simulink model "CellVoltageDiagnostics_HIL_Test_Automation"  (R2022b)
settings: Solver=FixedStepDiscrete  StartTime=0.0  StopTime=100  FixedStep=0.001  RelTol=1e-3  EnableMultiTasking=on
PreLoadFcn:
  | ts = 0.1
libraries: fl_lib x9, nesl_utility x9, speedgoatlib_IO133 x2, speedgoatlib_PIL x1, BatteryPack_lib x1
settings Model: DataDictionary=Shared_DD_TMS570.sldd  sg_rtwmakecfg_data=_sglibc__PIL_HWD__Pilpxi_  SimulationMode=external  Creator=cpatel  LastModifiedBy=mathieu.lu-dac
settings SolverCC: ConcurrentTasks=on  AlgebraicLoopSolver=TrustRegion  PositivePriorityOrder=on  AutoInsertRateTranBlk=on  InsertRTBMode=Never (minimum delay)
settings DataIOCC: SaveFormat=StructureWithTime  SaveOutput=off  SignalLogging=off  DSMLogging=off  SaveTime=off  SignalLoggingName=logsOut
settings OptimizationCC: BlockReduction=off  BooleanDataType=off  OptimizeBlockIOStorage=off  BufferReuse=off  GlobalBufferReuse=off  ExpressionFolding=off  LocalBlockOutputs=off  InitFltsAndDblsToZero=on  OptimizeDataStoreBuffers=off  BusAssignmentInplaceUpdate=off
settings DebuggingCC: SaveWithParameterizedLinksMsg=none  CheckExecutionContextPreStartOutputMsg=on  SignalResolutionControl=TryResolveAllWithWarning  TasksWithSamePriorityMsg=none  UnconnectedInputMsg=warning  UnconnectedOutputMsg=warning  UnconnectedLineMsg=warning  SFUnexpectedBacktrackingDiag=warning  SFNoUnconditionalDefaultTransitionDiag=warning  SFExecutionAtInitializationDiag=none  SFMachineParentedDataDiag=warning  ArithmeticOperatorsInVariantConditions=warning
settings HardwareCC: ProdBitPerLong=64  ProdLongLongMode=on  ProdHWDeviceType=Intel->x86-64 (Linux 64)
settings ModelReferenceCC: EnableRefExpFcnMdlSchedulingChecks=on  PropagateSignalLabelsOutOfModel=off
settings SFSimCC: SimUseLocalCustomCode=off  CustomCodeUndefinedFunction=UseInterfaceOnly
settings RTWCC: Description=Simulink Real-Time  SystemTargetFile=slrealtime.tlc  TemplateMakefile=slrealtime_default_tmf  RTWVerbose=off  RTWUseLocalCustomCode=off  Toolchain=Simulink Real-Time Toolchain  BuildConfiguration=Faster Runs  CodeExecutionProfiling=on  TargetLang=C++  DLArmComputeVersion=19.05
settings CodeAppCC: StateflowObjectComments=on
settings SimulinkRealTimeTargetCC: UseGCCFastMath=on
settings ConfigComp: CovMetricSettings=dw  CovSaveCumulativeToWorkspaceVar=on  CovSaveSingleToWorkspaceVar=on  CovExternalEMLEnable=off  CovSFcnEnable=off

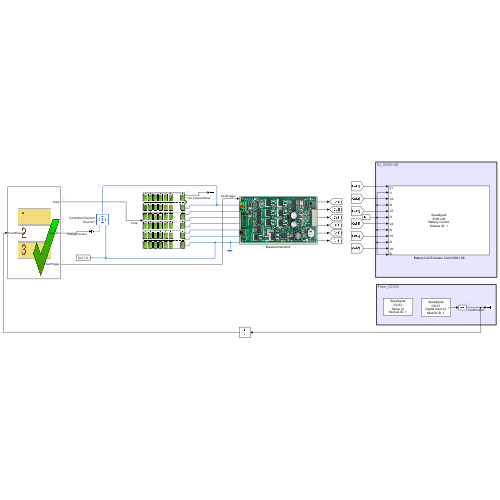
[thumbnail: Simulink's stored preview of the top-level diagram]
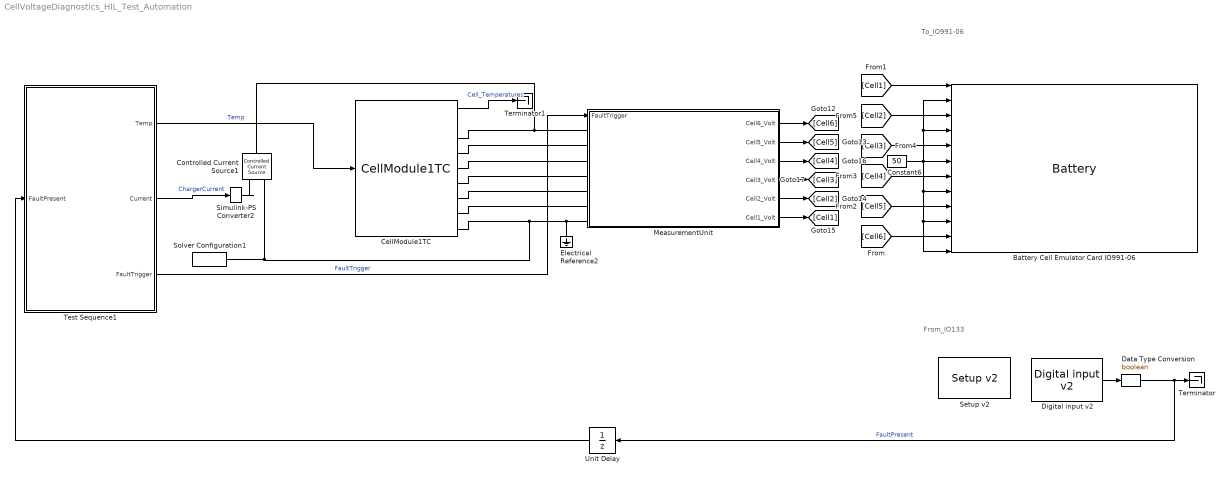
== system CellVoltageDiagnostics_HIL_Test_Automation ==
  note: To_IO991-06
  note: From_IO133
  Battery Cell Emulator Card IO991-06 : speedgoatlib_PIL/Battery  id=1  card_type=IO991-06 (6 channels, 0-7V output, 300mA source, 100mA sink)  channel_vector=[1,2,3,4,5,6]  init_enable_vector=ones(1,6)  reset_enable_vector=ones(1,6)  init_voltage_vector=3.6*ones(1,6)  reset_voltage_vector=ones(1,6)  init_current_vector=[0]  reset_current_vector=[0]  show_input_enable=off  show_output=off  ts=ts  slot=[6,15]  VendorID=0  SubVendorID=0  DeviceID=0  SubDeviceID=0  category=1  NumCh=0  MinVout=0  MaxVout=0  MinIsink=0  MaxIsink=0  mask(IOPIL_battery){}
      settings: SourceProductName=Simulink Real-Time: Speedgoat I/O Blockset
  CellModule1TC : BatteryPack_lib/CellModule1TC  SystemSampleTime=-1  VariantActivationTime=update diagram  Latency=0  AutoFrameSizeCalculation=off
      mask Display:
      | % This is a new mask on top of the base mask.
      | % Use "View base mask" link below to see the base mask.
      | image('BatteryPack.png');
  Constant6 : Constant  Value=50
  Controlled Current Source1 : fl_lib/Electrical/Electrical Sources/Controlled Current Source
      settings: LogSimulationData=on
  Data Type Conversion : DataTypeConversion  OutDataTypeStr=boolean  SaturateOnIntegerOverflow=off  RndMeth=Floor
  "Digital input v2 " : speedgoatlib_IO133/Digital input v2   parModuleId=1  parSampleTime=0.1  parPciSlot=-1  parDiChannels=1
      settings: SourceProductName=Simulink Real-Time: Speedgoat I/O Blockset
  Electrical Reference2 : fl_lib/Electrical/Electrical Elements/Electrical Reference
  MeasurementUnit : Subsystem
      mask Display: image('TCU.png');
  "Setup v2 " : speedgoatlib_IO133/Setup v2   parPciSlot=-1  parModuleId=1  parInterModuleSync=None  parConvClockBaseRate=20MHz  parConvClock1Divider=20000  parConvClock2Divider=20000  parFrameTriggerEnable=off  parFrameTriggerDivider=10  parConvClock1BaseRate=1  parConvClock2BaseRate=1  parFrameTriggerClock=1  parAdcChannels=[]  parAdcRange1=+-5V  parAdcRange2=+-5V  parAdcVoltageRange=[1 1]  parAdcOversampling1=None  parAdcOversampling2=None  parAdcOversamplRate=[1 1]  parAdcAutoCorrection=on  parAdcContSampling=off  parAdcDmaEnable=off  parAdcDmaClock=Clock 1  parAdcFrameSize_=100  parAdcSampleTime_=-1  parAdcActiveDmaDevices=[1 1]  parAdcFrameTriggerEnable=0  parAdcFrameSize=100  parAdcSampleTime=0.1  parDacChannels=[1]  parDacInitValues=0  parDacReset=1  parDacRange1=0-5V  parDacRange2=0-5V  parDacRange3=0-5V  parDacRange4=0-5V  parDacRange5=0-5V  parDacRange6=0-5V  parDacRange7=0-5V  parDacRange8=0-5V  parDacVoltageRange=[1 1 1 1 1 1 1 1]  parDacAutoCorrection=on  parDacSyncOut=on  parDacDmaEnable=off  parDacDmaLatency=Until next frame  parDacDmaClock=Clock 1  parDacFrameSize_=100  parDacSampleTime_=-1  parDacActiveDmaDevices=[1 1]  parDacFrameTriggerEnable=0  parDacFrameSize=100  parDacSampleTime=0.1  parDoChannels=[]  parDoInitValues=0  parDoReset=0  parDiChannels=[1]  parDiDebounceEnable=off  parDiDebounceTime=0  parDiDebounceValue=0  parDioPullRefFront=Pull-up 3.3V  parDioPullRefRear=Floating
      settings: SourceProductName=Simulink Real-Time: Speedgoat I/O Blockset
  Simulink-PS Converter2 : nesl_utility/Simulink-PS Converter  PhysicalDomain=network_engine_domain  SubClassName=ps_input  LeftPortType=input  RightPortType=output  PseudoPeriodic=off  Frequencies=[]  NoiseDistribution=none  NoiseParameters=[]  Unit=1  AffineConversion=off  FilteringAndDerivatives=zero  SimscapeFilterOrder=1  InputFilterTimeConstant=0.001  UdotUserProvided=1
  Solver Configuration1 : nesl_utility/Solver Configuration  PhysicalDomain=network_engine_domain  SubClassName=solver  LeftPortType=input  RightPortType=generic  Tones=[]  Harmonics=[]  SimulateNoise=off  Profile=off  UseLocalSampling=off  EnableSwitchedLinearOptims=on  FrequencyDomain=off  UseCCode=off  RelTol=0.001  AbsTol=1e-06  MinStep=1e-09  ToWorkspace=off  RevertToSquareIcSolve=off  NumHomotopyIterations=100  PhasorMode=off  PhasorModeNumHarmonics=1  ConsistencySolver=NEWTON_FTOL  IndexReductionMethod=DerivativeReplacement  DoDC=off  ResidualTolerance=1e-09  ConsistencyTolSource=GLOBAL  ConsistencyAbsTol=0.001  ConsistencyRelTol=0.001  ConsistencyTolFactor=0.001  UseLocalSolver=on  LocalSolverChoice=NE_BACKWARD_EULER_ADVANCER  ResolveIndetEquations=on  FunctionEvalNumThread=1  LocalSolverSampleTime=ts  DoFixedCost=on  MaxNonlinIter=3  MaxModeIter=2  ComputeImpulses=off  ImpulseIterations=2  LinearAlgebra=auto  LinearAlgebraNumThread=0  EquationFormulation=NE_TIME_EF  DelaysMemoryBudget=1024  AutomaticFiltering=off  FilteringTimeConstant=0.001  PartitionStorageMethod=AS_NEEDED  PartitionMemoryBudget=1024  PartitionMethod=FAST
  Terminator : Terminator
  Terminator1 : Terminator
  Test Sequence1 : Test Sequence  TreatAsAtomicUnit=on
  Unit Delay : UnitDelay  SampleTime=-1  HasFrameUpgradeWarning=on
  wires:
  Data Type Conversion/1 -> Unit Delay/1, Terminator/1  "FaultPresent"
  "Digital input v2 "/1 -> Data Type Conversion/1
  Constant6/1 -> Battery Cell Emulator Card IO991-06/2, Battery Cell Emulator Card IO991-06/4, Battery Cell Emulator Card IO991-06/6, Battery Cell Emulator Card IO991-06/12, Battery Cell Emulator Card IO991-06/10, Battery Cell Emulator Card IO991-06/8
  [Cell6] -> Battery Cell Emulator Card IO991-06/11
  [Cell1] -> Battery Cell Emulator Card IO991-06/1
  [Cell5] -> Battery Cell Emulator Card IO991-06/9
  [Cell4] -> Battery Cell Emulator Card IO991-06/7
  [Cell3] -> Battery Cell Emulator Card IO991-06/5
  [Cell2] -> Battery Cell Emulator Card IO991-06/3
  Unit Delay/1 -> Test Sequence1/1(FaultPresent)
  MeasurementUnit/6(Cell1_Volt) -> [Cell1]
  MeasurementUnit/5(Cell2_Volt) -> [Cell2]
  CellModule1TC/1 -> Terminator1/1  "Cell_Temperatures"
  MeasurementUnit/3(Cell4_Volt) -> [Cell4]
  Test Sequence1/3(FaultTrigger) -> MeasurementUnit/1(FaultTrigger)  "FaultTrigger"
  Test Sequence1/2(Current) -> Simulink-PS Converter2/1  "ChargerCurrent"
  MeasurementUnit/2(Cell5_Volt) -> [Cell5]
  Test Sequence1/1(Temp) -> CellModule1TC/1  "Temp"
  MeasurementUnit/1(Cell6_Volt) -> [Cell6]
  MeasurementUnit/4(Cell3_Volt) -> [Cell3]
  connections:
  CellModule1TC/RConn7 -- Solver Configuration1/RConn1 -- Controlled Current Source1/RConn2 -- Electrical Reference2/LConn1 -- MeasurementUnit/LConn7
  MeasurementUnit/LConn1 -- CellModule1TC/RConn1 -- Controlled Current Source1/LConn1
  CellModule1TC/RConn4 -- MeasurementUnit/LConn4
  CellModule1TC/RConn3 -- MeasurementUnit/LConn3
  CellModule1TC/RConn6 -- MeasurementUnit/LConn6
  Simulink-PS Converter2/RConn1 -- Controlled Current Source1/RConn1
  CellModule1TC/RConn2 -- MeasurementUnit/LConn2
  CellModule1TC/RConn5 -- MeasurementUnit/LConn5

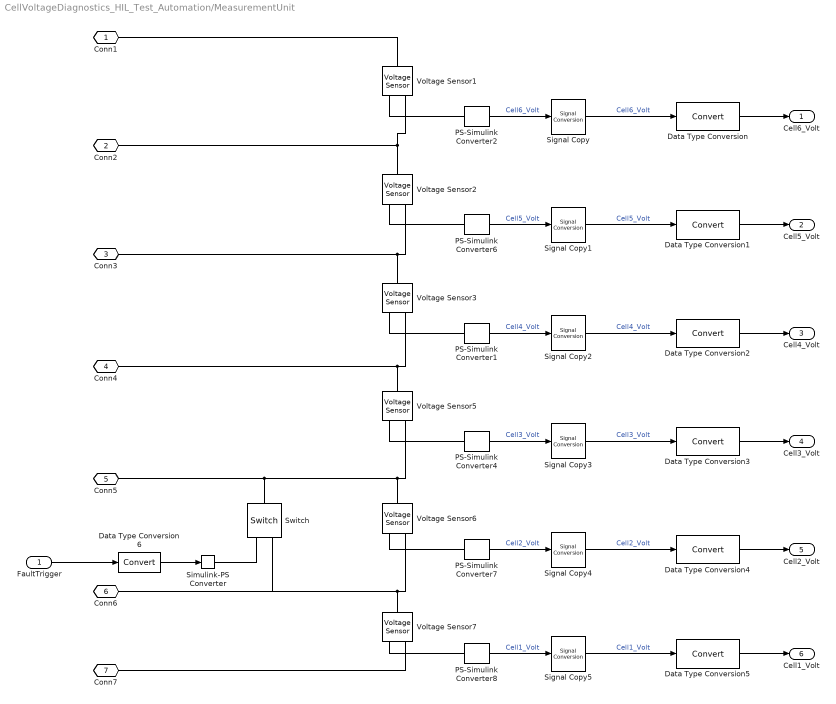
== system CellVoltageDiagnostics_HIL_Test_Automation/MeasurementUnit ==
  FaultTrigger : Inport
  Data Type Conversion{,1..6} (7 alike) : DataTypeConversion  SaturateOnIntegerOverflow=off  RndMeth=Floor
  PS-Simulink Converter{1..2,4,6..8} (6 alike) : nesl_utility/PS-Simulink Converter  PhysicalDomain=network_engine_domain  SubClassName=ps_output  LeftPortType=input  RightPortType=output  PseudoPeriodic=off  Frequencies=[]  VectorFormat=1-D array  Unit=V  AffineConversion=off
  Signal Copy{,1..5} (6 alike) : SignalConversion  OverrideOpt=off
  Simulink-PS Converter : nesl_utility/Simulink-PS Converter  PhysicalDomain=network_engine_domain  SubClassName=ps_input  LeftPortType=input  RightPortType=output  PseudoPeriodic=off  Frequencies=[]  NoiseDistribution=none  NoiseParameters=[]  Unit=1  AffineConversion=off  FilteringAndDerivatives=provide  SimscapeFilterOrder=1  InputFilterTimeConstant=0.001  UdotUserProvided=0
  Switch : fl_lib/Electrical/Electrical Elements/Switch  R_closed=0.01 Ohm  G_open=1e-8 1/Ohm  Threshold=0.5  i_specify=off  i_priority=None  i=0 A  i_nominal_specify=off  i_nominal_unit=A  i_nominal_value=1  v_specify=off  v_priority=None  v=0 V  v_nominal_specify=off  v_nominal_unit=V  v_nominal_value=1
  Voltage Sensor{1..3,5..7} (6 alike) : fl_lib/Electrical/Electrical Sensors/Voltage Sensor
  Conn1 : PMIOPort  Side=Left
  Conn2 : PMIOPort  Port=2  Side=Left
  Conn3 : PMIOPort  Port=3  Side=Left
  Conn4 : PMIOPort  Port=4  Side=Left
  Conn5 : PMIOPort  Port=5  Side=Left
  Conn6 : PMIOPort  Port=6  Side=Left
  Conn7 : PMIOPort  Port=7  Side=Left
  Cell6_Volt : Outport  VectorParamsAs1DForOutWhenUnconnected=off
  Cell5_Volt : Outport  Port=2  VectorParamsAs1DForOutWhenUnconnected=off
  Cell4_Volt : Outport  Port=3  VectorParamsAs1DForOutWhenUnconnected=off
  Cell3_Volt : Outport  Port=4  VectorParamsAs1DForOutWhenUnconnected=off
  Cell2_Volt : Outport  Port=5  VectorParamsAs1DForOutWhenUnconnected=off
  Cell1_Volt : Outport  Port=6  VectorParamsAs1DForOutWhenUnconnected=off
  wires:
  PS-Simulink Converter1/1 -> Signal Copy2/1  "Cell4_Volt"
  PS-Simulink Converter7/1 -> Signal Copy4/1  "Cell2_Volt"
  PS-Simulink Converter2/1 -> Signal Copy/1  "Cell6_Volt"
  PS-Simulink Converter4/1 -> Signal Copy3/1  "Cell3_Volt"
  PS-Simulink Converter8/1 -> Signal Copy5/1  "Cell1_Volt"
  PS-Simulink Converter6/1 -> Signal Copy1/1  "Cell5_Volt"
  Data Type Conversion/1 -> Cell6_Volt/1
  Data Type Conversion1/1 -> Cell5_Volt/1
  Data Type Conversion2/1 -> Cell4_Volt/1
  Data Type Conversion3/1 -> Cell3_Volt/1
  Data Type Conversion5/1 -> Cell1_Volt/1
  Data Type Conversion4/1 -> Cell2_Volt/1
  FaultTrigger/1 -> Data Type Conversion6/1
  Data Type Conversion6/1 -> Simulink-PS Converter/1
  Signal Copy/1 -> Data Type Conversion/1  "Cell6_Volt"
  Signal Copy1/1 -> Data Type Conversion1/1  "Cell5_Volt"
  Signal Copy2/1 -> Data Type Conversion2/1  "Cell4_Volt"
  Signal Copy3/1 -> Data Type Conversion3/1  "Cell3_Volt"
  Signal Copy4/1 -> Data Type Conversion4/1  "Cell2_Volt"
  Signal Copy5/1 -> Data Type Conversion5/1  "Cell1_Volt"
  connections:
  PS-Simulink Converter2/LConn1 -- Voltage Sensor1/RConn1
  Voltage Sensor2/LConn1 -- Voltage Sensor1/RConn2 -- Conn2/RConn1
  Voltage Sensor6/RConn2 -- Voltage Sensor7/LConn1 -- Conn6/RConn1 -- Switch/RConn2
  Voltage Sensor5/RConn1 -- PS-Simulink Converter4/LConn1
  Voltage Sensor7/RConn1 -- PS-Simulink Converter8/LConn1
  Voltage Sensor5/LConn1 -- Voltage Sensor3/RConn2 -- Conn4/RConn1
  Conn5/RConn1 -- Voltage Sensor6/LConn1 -- Voltage Sensor5/RConn2 -- Switch/LConn1
  Voltage Sensor3/LConn1 -- Voltage Sensor2/RConn2 -- Conn3/RConn1
  Voltage Sensor6/RConn1 -- PS-Simulink Converter7/LConn1
  Voltage Sensor2/RConn1 -- PS-Simulink Converter6/LConn1
  Voltage Sensor3/RConn1 -- PS-Simulink Converter1/LConn1
  Voltage Sensor1/LConn1 -- Conn1/RConn1
  Voltage Sensor7/RConn2 -- Conn7/RConn1
  Switch/RConn1 -- Simulink-PS Converter/RConn1

== stateflow chart CellVoltageDiagnostics_HIL_Test_Automation/Test Sequence1 ==
  state Init
    Temp = 295;
    Current = 0;
    FaultTrigger = 0;
  state TestCase1
    Temp = 295;
    Current = 0;
    FaultTrigger = 0;
    state step_1_1
      Current = 20;
      verify(FaultPresent == true,'Battery Fault Due to OverVoltage')
    state step_1_2
      Current = -20
      verify(FaultPresent == false,'Battery Fault Due to UnderVoltage')
    (default) -> step_1_1
    step_1_1 -> step_1_2 : [after(5,sec)
        | ]
  state TestCase2
    Temp = 295;
    Current = -20;
    FaultTrigger = 0;
    state step_6
      FaultTrigger = 1;
      verify(FaultPresent == false,'Battery Fault Due to Short Terminal')
    state step_7
      verify(FaultPresent == true,'Battery Fault Due to Short Terminal')
    (default) -> step_6
    step_6 -> step_7 : [
        | after(1,sec)
        | ]
  (default) -> Init
  Init -> (junction 109) [order 2] : [TestCase == 2
      | ]
  (junction 109) -> (junction 73)
  Init -> TestCase1 [order 1] : [TestCase == 1
      | ]
  (junction 73) -> TestCase2
  data: Temp output; Current output; FaultTrigger output; FaultPresent input; TestCase parameter
